simulink model "RobotX_ss_acoustics_1020"  (R2014a)
settings: Solver=FixedStepDiscrete  StartTime=0.0  StopTime=inf  FixedStep=.25  RelTol=1e-3
undefined symbols (not defined in the file): Com1, Com3, DiscIntNeverNeededParam, standard
libraries: xpcseriallib x19, dspmtrx3 x3, slrtlib x3, simulink x2, speedgoatlib x1, speedgoatlib_IO102 x1
(part 3 of 3)

== matlab function RobotX_ss_acoustics_1020/Main FSM/Acoustic FSM/Move 2/GPSMove ==
  data: GoalNED input; X input; Finished output; valid output; Y input; Psi input; pts output
function [Finished,valid,pts] = GPSmove(GoalNED,X,Y,Psi)
%Written by Dylan DeGaetano on September 1, 2014
%Last edited by: Anderson Lebbad
%
%This function will go to a given NED cooridnate, last edit changed the
%goal pt and variable names

persistent Sample
if isempty(Sample)
Sample = 0;
end
Finished = 0;
pts = zeros(8,2);
%$Distance to object in meters
if Sample >= 100
    Sample = 0;
end

if Sample == 0
    pts(1,1) = X+5*cos(Psi*pi/180);
    pts(1,2) = Y+5*cos(Psi*pi/180);
    pts(8,1) = GoalNED(1,1);
    pts(8,2) = GoalNED(1,2);
    pts(2,:) = pts(1,:) +(1*(GoalNED-pts(1,:))/7);
    pts(3,:) = pts(1,:) +(2*(GoalNED-pts(1,:))/7);
    pts(4,:) = pts(1,:) +(3*(GoalNED-pts(1,:))/7);
    pts(5,:) = pts(1,:) +(4*(GoalNED-pts(1,:))/7);
    pts(6,:) = pts(1,:) +(5*(GoalNED-pts(1,:))/7);
    pts(7,:) = pts(1,:) +(6*(GoalNED-pts(1,:))/7);
    Sample = 1; 
    valid = 1;
    
else 
    range = sqrt(sum((GoalNED - [X Y]).^2));
    if range <= 5
        Finished = 1;
    end
    valid = 0;
    Sample = Sample + 1;
end

== matlab function RobotX_ss_acoustics_1020/Main FSM/Acoustic FSM/Move 3/CalcTimes ==
  data: pts input; u input; Data output
function Data = calcTimes(pts, u)
%Written by Anderson Lebbad on August 9, 2014
%Last Edited: Dylan DeGaetano September 1, 2014

%Calculates times for the boat to get to points for a trajectory, and
%formats Data for communication

%Initialize
Data = zeros(24,1);
traj = zeros(8,3);
traj(:,1:2) = pts;



for k = 2:8
    %Calculate distance to travel from last point
    distTravel = sqrt(sum((pts(k-1,:)-pts(k,:)).^2));
    %Assume 1m per second speed
    traj(k,3) = traj(k-1,3) + distTravel;
    %Add time based off initial velocity to get to first point past initial
    if k == 2
        traj(k,3) = traj(k,3) + 2.5*abs(2-u);
    end
end


%Output Data
for i=1:8
    for j = 1:3
        Data(3*(i-1)+j) = traj(i,j);
    end
end

== matlab function RobotX_ss_acoustics_1020/Main FSM/Acoustic FSM/Move 3/GPSMove ==
  data: GoalNED input; X input; Finished output; valid output; Y input; Psi input; pts output
function [Finished,valid,pts] = GPSmove(GoalNED,X,Y,Psi)
%Written by Dylan DeGaetano on September 1, 2014
%Last edited by: Anderson Lebbad
%
%This function will go to a given NED cooridnate, last edit changed the
%goal pt and variable names

persistent Sample
if isempty(Sample)
Sample = 0;
end
Finished = 0;
pts = zeros(8,2);
%$Distance to object in meters
if Sample >= 100
    Sample = 0;
end

if Sample == 0
    pts(1,1) = X+5*cos(Psi*pi/180);
    pts(1,2) = Y+5*cos(Psi*pi/180);
    pts(8,1) = GoalNED(1,1);
    pts(8,2) = GoalNED(1,2);
    pts(2,:) = pts(1,:) +(1*(GoalNED-pts(1,:))/7);
    pts(3,:) = pts(1,:) +(2*(GoalNED-pts(1,:))/7);
    pts(4,:) = pts(1,:) +(3*(GoalNED-pts(1,:))/7);
    pts(5,:) = pts(1,:) +(4*(GoalNED-pts(1,:))/7);
    pts(6,:) = pts(1,:) +(5*(GoalNED-pts(1,:))/7);
    pts(7,:) = pts(1,:) +(6*(GoalNED-pts(1,:))/7);
    Sample = 1; 
    valid = 1;
    
else 
    range = sqrt(sum((GoalNED - [X Y]).^2));
    if range <= 5
        Finished = 1;
    end
    valid = 0;
    Sample = Sample + 1;
end

== matlab function RobotX_ss_acoustics_1020/Main FSM/Start//Speedgate/GPS Move/LLA to NED ==
  data: GoalLLA input; GoalNED output; NED_origin input
function GoalNED = LLA2NEDfun(GoalLLA,NED_origin)
%Written by Anderson Lebbad on September 20, 2014
%Last edited by:
%
%This function converts a target Latitude, Longitude, Altitude (LLA) point
%into North, East, Down (NED) coordinates

%First convert to earth centered, earth fixed frame
GoalECEF = lla2ecef([GoalLLA*(pi/180), 0]');
%Then convert from ECEF to North East Down
GoalNEDvect = ecef2ned(NED_origin'*(pi/180),GoalECEF);
GoalNED = GoalNEDvect(1:2)';

end

function x_ecef = lla2ecef(x_lla)
% LLE2ECEF: Converts from geodetic latitude, longitude, and altitude to earth-centered earth-fixed Cartesian coordinates
% INPUT: latitude phi (rad), longitude lambda (rad), altitude h (m)
% OUTPUT: [x, y, z]' (m) earth-centered earth-fixed Cartesian coordinates
    a = 6378137; % equatorial radius of ellipsoid (semi-major axis) (m)
    b = 6356752; % polar axis radius of ellipsoid (semi-minor axis) (m)

    phi = x_lla(1);
    lambda = x_lla(2);
    h = x_lla(3);
    
    % auxiliar quantities f, e, and N
    f = (a-b)/a;
    e = f*(2-f);
    N = a/sqrt(1-(e*sin(phi))^2);
    x_ecef = [(N+h)*cos(phi)*cos(lambda); (N+h)*cos(phi)*sin(lambda); (N*(1-e^2)+h)*sin(phi)];
end

function [x_ned] = ecef2ned(ned_lla, x_ecef)
% ECEF2NED Converts from earth-centered, earth-fixed Cartesian coordinates to tangent plane
% INPUT:
% 1) x_ecef=[x,y,z]' (m) earth-centered, earth-fixed Cartesian coordinates
% 2) ned_lla=[phi,lambda]' consiting of latitude phi (rad), longitude lambda (rad) of NED origin
% OUTPUT:
% 1) x_ned=[x,y,z]' (m) in NED coordinate system with the origin [phi,lambda]'

    phi = ned_lla(1);
    lambda = ned_lla(2);

    % transformation  matrix
    T = [-sin(phi)*cos(lambda) -sin(phi)*sin(lambda)  cos(phi)
         -sin(lambda)           cos(lambda)           0
          cos(phi)*cos(lambda)   cos(phi)*sin(lambda)  sin(phi)];

     x_ned = T*(x_ecef-lla2ecef([phi, lambda, 0]')); % convert to NED
     x_ned(3) = -x_ned(3);
end

== matlab function RobotX_ss_acoustics_1020/Sensors/Serial In/MATLAB Function3 ==
  data: Time input; asciiHRT output; Lat input; Long input; Mode input; Task input
% This function creates the heartbeat message to be sent from Speedgoat in
% ascii code
% Written by: Edward Zhu
% Date: 9/17/14

function asciiHRT = asciiHRTEncoder(Time, Lat, Long, Mode, Task)

% Initialize output message vector as the serial output block expects 128
% character message
asciiHRT = uint8(zeros(1,128));

% Convert static strings to ascii code
asciiMsgID = uint8('$RXHRT,');
asciiComma = uint8(',');
asciiDeciPt = uint8('.');
if Lat >= 0
    asciiNS = uint8('N,');
else
    Lat = -Lat;
    asciiNS = uint8('S,');
end
if Long >= 0
    asciiEW = uint8('E,');
else
    Long = -Long;
    asciiEW = uint8('W,');
end
asciiTeamID = uint8('FAUVU,');
asciiMsgEnd = uint8('*');
asciiMsgCRLF = [13 10];

% Convert UTC Time input (hhmmss) into ascii code
asciiTime = uint8(zeros(1,7));
asciiTime(7) = asciiComma;

for timeChar = 1:6
    asciiTime(timeChar) = floor(mod(Time,10^(7-timeChar))/...
        10^(6-timeChar)) + 48;
end

% Convert latitude (dd.mmmmmm) into ascii code
asciiLat = uint8(zeros(1,10));
asciiLat(10) = asciiComma;
asciiLat(3) = asciiDeciPt;

latInt = floor(Lat);
for latIntChar = 1:2
    asciiLat(latIntChar) = floor(mod(latInt,10^(3-latIntChar))/...
        10^(2-latIntChar)) + 48;
end

latDeci = mod(Lat,latInt) * 10^6;
for latDeciChar = 1:6
    asciiLat(latDeciChar+3) = floor(mod(latDeci,10^(7-latDeciChar))/...
        10^(6-latDeciChar)) + 48;
end

% Convert longitude (ddd.mmmmmm) into ascii code
asciiLong = uint8(zeros(1,11));
asciiLong(11) = asciiComma;
asciiLong(4) = asciiDeciPt;

longInt = floor(Long);
for longIntChar = 1:3
    asciiLong(longIntChar) = floor(mod(longInt,10^(4-longIntChar))/...
        10^(3-longIntChar)) + 48;
end

longDeci = mod(Long,longInt) * 10^6;
for longDeciChar = 1:6
    asciiLong(longDeciChar+4) = floor(mod(longDeci,10^(7-longDeciChar))/...
        10^(6-longDeciChar)) + 48;
end

% Convert vehicle mode into ascii (1 = RC, 2 = Auto)
if Mode ~= 1 || Mode ~= 2
    Mode = 1;
    asciiMode = [uint8(Mode+48) asciiComma];
else
    asciiMode = [uint8(Mode+48) asciiComma];
end

% Convert vehicle task into ascii
asciiTask = [uint8(Task+48) asciiMsgEnd];

% Concat individual ascii arrays into one array
asciiPreChkSum = cat(2,asciiMsgID,asciiTime,asciiLat,asciiNS,asciiLong,asciiEW,...
    asciiTeamID,asciiMode,asciiTask);

% Calculate the checksum of the message from the '$' to the '*' and convert
% to hex
chkSum = uint8(0);

for chksumChar = 1:(length(asciiPreChkSum)-2)
    chkSum = bitxor(chkSum,asciiPreChkSum(chksumChar+1));
end

% Convert the checksum to ascii
chkSum = dec2hex(chkSum);
asciiChkSum = uint8(zeros(1,length(chkSum))+32);
for i = 1:length(chkSum)
    asciiChkSum(i) = uint8(chkSum(i));
end

% Concat the checksum and the '/r/n' to the end of the message
asciiPostChkSum = cat(2,asciiPreChkSum,asciiChkSum,asciiMsgCRLF);

% Output the final message
asciiHRT(1:length(asciiPostChkSum)) = asciiPostChkSum;

== matlab function RobotX_ss_acoustics_1020/Sensors/Serial In/Data Update1 ==
  data: Valid input; ControlMode input; V output; C output; L output; A output; Data input; D1 output; D2 output; D3 output; D4 output; D5 output; D6 output; D7 output; D8 output; D9 output; D10 output; D11 output; D12 output; D13 output; D14 output; D15 output; D16 output; D17 output; D18 output; D19 output; D20 output; D21 output; D22 output; D23 output; D24 output; Activate input
function [V,C,L,A,D1,D2,D3,D4,D5,D6,D7,D8,D9,D10,D11,D12,D13,D14,D15,D16,D17,...
    D18,D19,D20,D21,D22,D23,D24] = dataSplit(Valid,ControlMode,Data,Activate)
%Written by Anderson Lebbad on August 10, 2014
%Last Edited by: Anderson Lebbad on September 11, 2014

%This function splits the data vector into the twelve channels it is
%composed of for communication

persistent HoldData

A = Activate;

if isempty(HoldData)
    HoldData = zeros(26,1);
end

L = 8;

if Valid == 1
    HoldData(1) = Valid;
    HoldData(2) = ControlMode;
    HoldData(3) = Data(1);
    HoldData(4) = Data(2);
    HoldData(5) = Data(3);
    HoldData(6) = Data(4);
    HoldData(7) = Data(5);
    HoldData(8) = Data(6);
    HoldData(9) = Data(7);
    HoldData(10) = Data(8);
    HoldData(11) = Data(9);
    HoldData(12) = Data(10);
    HoldData(13) = Data(11);
    HoldData(14) = Data(12);
    HoldData(15) = Data(13);
    HoldData(16) = Data(14);
    HoldData(17) = Data(15);
    HoldData(18) = Data(16);
    HoldData(19) = Data(17);
    HoldData(20) = Data(18);
    HoldData(21) = Data(19);
    HoldData(22) = Data(20);
    HoldData(23) = Data(21);
    HoldData(24) = Data(22);
    HoldData(25) = Data(23);
    HoldData(26) = Data(24);
end

V = HoldData(1);
C = HoldData(2);
D1 = HoldData(3);
D2 = HoldData(4);
D3 = HoldData(5);
D4 = HoldData(6);
D5 = HoldData(7);
D6 = HoldData(8);
D7 = HoldData(9);
D8 = HoldData(10);
D9 = HoldData(11);
D10 = HoldData(12);
D11 = HoldData(13);
D12 = HoldData(14);
D13 = HoldData(15);
D14 = HoldData(16);
D15 = HoldData(17);
D16 = HoldData(18);
D17 = HoldData(19);
D18 = HoldData(20);
D19 = HoldData(21);
D20 = HoldData(22);
D21 = HoldData(23);
D22 = HoldData(24);
D23 = HoldData(25);
D24 = HoldData(26);

end

== matlab function RobotX_ss_acoustics_1020/Main FSM/Acoustic FSM/Main Enabler ==
  data: taskSelector output; Drive1En output; Acoustic1En output; Drive2En output; Drive1Fin input; Acoustic1Fin input; Drive2Fin input; Acoustic2Fin input; Drive3Fin input; Acoustic3Fin input; Acoustic2En output; Drive3En output; Acoustic3En output; PointEn output
function [taskSelector,Drive1En,Acoustic1En,Drive2En,Acoustic2En,Drive3En,...
    Acoustic3En,PointEn] = taskEnabler(Drive1Fin,Acoustic1Fin,Drive2Fin,...
    Acoustic2Fin,Drive3Fin,Acoustic3Fin)
%Written by Anderson Lebbad on July 19, 2013
%Last Edited: Edward Zhu on June 2, 2014
%   Substring search for task was written in
%   Case switches were redundant, combined with first set of if statements

%Changes the value of MainMode and the enablers for the tasks within the
%Main FSM.

% Initialize enable signals
Drive1En = 0;
Acoustic1En = 0;
Drive2En = 0;
Acoustic2En = 0;
Drive3En = 0;
Acoustic3En = 0;
PointEn = 0;

% Set enable signals based on state completion
if Drive1Fin == 0
    Drive1En = 1;
    taskSelector = 1;
elseif Acoustic1Fin == 0
    Acoustic1En = 1;
    taskSelector = 2;
elseif Drive2Fin == 0
    Drive2En = 1;
    taskSelector = 3;
elseif Acoustic2Fin == 0
    Acoustic2En = 1;
    taskSelector = 4;
elseif Drive3Fin == 0
    Drive3En = 1;
    taskSelector = 5;
elseif Acoustic3Fin == 0
    Acoustic3En = 1;
    taskSelector = 6;
else
    PointEn = 1;
    taskSelector = 7;
end

== matlab function RobotX_ss_acoustics_1020/Main FSM/Acoustic FSM/Move 1/CalcTimes ==
  data: pts input; u input; Data output
function Data = calcTimes(pts, u)
%Written by Anderson Lebbad on August 9, 2014
%Last Edited: Dylan DeGaetano September 1, 2014

%Calculates times for the boat to get to points for a trajectory, and
%formats Data for communication

%Initialize
Data = zeros(24,1);
traj = zeros(8,3);
traj(:,1:2) = pts;



for k = 2:8
    %Calculate distance to travel from last point
    distTravel = sqrt(sum((pts(k-1,:)-pts(k,:)).^2));
    %Assume 1m per second speed
    traj(k,3) = traj(k-1,3) + distTravel;
    %Add time based off initial velocity to get to first point past initial
    if k == 2
        traj(k,3) = traj(k,3) + 2.5*abs(2-u);
    end
end


%Output Data
for i=1:8
    for j = 1:3
        Data(3*(i-1)+j) = traj(i,j);
    end
end

== matlab function RobotX_ss_acoustics_1020/Main FSM/Acoustic FSM/Move 1/GPSMove ==
  data: GoalNED input; X input; Finished output; valid output; Y input; Psi input; pts output
function [Finished,valid,pts] = GPSmove(GoalNED,X,Y,Psi)
%Written by Dylan DeGaetano on September 1, 2014
%Last edited by: Anderson Lebbad
%
%This function will go to a given NED cooridnate, last edit changed the
%goal pt and variable names

persistent Sample
if isempty(Sample)
Sample = 0;
end
Finished = 0;
pts = zeros(8,2);
%$Distance to object in meters
if Sample >= 100
    Sample = 0;
end

if Sample == 0
    pts(1,1) = X+5*cos(Psi*pi/180);
    pts(1,2) = Y+5*cos(Psi*pi/180);
    pts(8,1) = GoalNED(1,1);
    pts(8,2) = GoalNED(1,2);
    pts(2,:) = pts(1,:) +(1*(GoalNED-pts(1,:))/7);
    pts(3,:) = pts(1,:) +(2*(GoalNED-pts(1,:))/7);
    pts(4,:) = pts(1,:) +(3*(GoalNED-pts(1,:))/7);
    pts(5,:) = pts(1,:) +(4*(GoalNED-pts(1,:))/7);
    pts(6,:) = pts(1,:) +(5*(GoalNED-pts(1,:))/7);
    pts(7,:) = pts(1,:) +(6*(GoalNED-pts(1,:))/7);
    Sample = 1; 
    valid = 1;
    
else 
    range = sqrt(sum((GoalNED - [X Y]).^2));
    if range <= 5
        Finished = 1;
    end
    valid = 0;
    Sample = Sample + 1;
end

== matlab function RobotX_ss_acoustics_1020/Main FSM/Start//Speedgate/entrance/CalcTimes ==
  data: pts input; u input; Data output
function Data = calcTimes(pts, u)
%Written by Anderson Lebbad on August 9, 2014
%Last Edited: Dylan DeGaetano September 1, 2014

%Calculates times for the boat to get to points for a trajectory, and
%formats Data for communication

%Initialize
Data = zeros(24,1);
traj = zeros(8,3);
traj(:,1:2) = pts;



for k = 2:8
    %Calculate distance to travel from last point
    distTravel = sqrt(sum((pts(k-1,:)-pts(k,:)).^2));
    %Assume 1m per second speed
    traj(k,3) = traj(k-1,3) + distTravel;
    %Add time based off initial velocity to get to first point past initial
    if k == 2
        traj(k,3) = traj(k,3) + 2.5*abs(2-u);
    end
end


%Output Data
for i=1:8
    for j = 1:3
        Data(3*(i-1)+j) = traj(i,j);
    end
end

== matlab function RobotX_ss_acoustics_1020/Main FSM/Start//Speedgate/entrance/GPSMove ==
  data: GoalNED input; X input; Finished output; valid output; Y input; Psi input; pts output
function [Finished,valid,pts] = GPSmove(GoalNED,X,Y,Psi)
%Written by Dylan DeGaetano on September 1, 2014
%Last edited by: Anderson Lebbad
%
%This function will go to a given NED cooridnate, last edit changed the
%goal pt and variable names

persistent Sample
if isempty(Sample)
Sample = 0;
end
Finished = 0;
pts = zeros(8,2);
%$Distance to object in meters
if Sample >= 100
    Sample = 0;
end

if Sample == 0
    pts(1,1) = X+5*cos(Psi*pi/180);
    pts(1,2) = Y+5*cos(Psi*pi/180);
    pts(8,1) = GoalNED(1,1);
    pts(8,2) = GoalNED(1,2);
    pts(2,:) = pts(1,:) +(1*(GoalNED-pts(1,:))/7);
    pts(3,:) = pts(1,:) +(2*(GoalNED-pts(1,:))/7);
    pts(4,:) = pts(1,:) +(3*(GoalNED-pts(1,:))/7);
    pts(5,:) = pts(1,:) +(4*(GoalNED-pts(1,:))/7);
    pts(6,:) = pts(1,:) +(5*(GoalNED-pts(1,:))/7);
    pts(7,:) = pts(1,:) +(6*(GoalNED-pts(1,:))/7);
    Sample = 1; 
    valid = 1;
    
else 
    range = sqrt(sum((GoalNED - [X Y]).^2));
    if range <= 8
        Finished = 1;
    end
    valid = 0;
    Sample = Sample + 1;
end

== matlab function RobotX_ss_acoustics_1020/Main FSM/Start//Speedgate/exit/CalcTimes ==
  data: pts input; u input; Data output
function Data = calcTimes(pts, u)
%Written by Anderson Lebbad on August 9, 2014
%Last Edited: Dylan DeGaetano September 1, 2014

%Calculates times for the boat to get to points for a trajectory, and
%formats Data for communication

%Initialize
Data = zeros(24,1);
traj = zeros(8,3);
traj(:,1:2) = pts;



for k = 2:8
    %Calculate distance to travel from last point
    distTravel = sqrt(sum((pts(k-1,:)-pts(k,:)).^2));
    %Assume 1m per second speed
    traj(k,3) = traj(k-1,3) + distTravel;
    %Add time based off initial velocity to get to first point past initial
    if k == 2
        traj(k,3) = traj(k,3) + 2.5*abs(2-u);
    end
end


%Output Data
for i=1:8
    for j = 1:3
        Data(3*(i-1)+j) = traj(i,j);
    end
end

== matlab function RobotX_ss_acoustics_1020/Main FSM/Start//Speedgate/exit/GPSMove ==
  data: GoalNED input; X input; Finished output; valid output; Y input; Psi input; pts output
function [Finished,valid,pts] = GPSmove(GoalNED,X,Y,Psi)
%Written by Dylan DeGaetano on September 1, 2014
%Last edited by: Anderson Lebbad
%
%This function will go to a given NED cooridnate, last edit changed the
%goal pt and variable names

persistent Sample
if isempty(Sample)
Sample = 0;
end
Finished = 0;
pts = zeros(8,2);
%$Distance to object in meters
if Sample >= 100
    Sample = 0;
end

if Sample == 0
    pts(1,1) = X+5*cos(Psi*pi/180);
    pts(1,2) = Y+5*cos(Psi*pi/180);
    pts(8,1) = GoalNED(1,1);
    pts(8,2) = GoalNED(1,2);
    pts(2,:) = pts(1,:) +(1*(GoalNED-pts(1,:))/7);
    pts(3,:) = pts(1,:) +(2*(GoalNED-pts(1,:))/7);
    pts(4,:) = pts(1,:) +(3*(GoalNED-pts(1,:))/7);
    pts(5,:) = pts(1,:) +(4*(GoalNED-pts(1,:))/7);
    pts(6,:) = pts(1,:) +(5*(GoalNED-pts(1,:))/7);
    pts(7,:) = pts(1,:) +(6*(GoalNED-pts(1,:))/7);
    Sample = 1; 
    valid = 1;
    
else 
    range = sqrt(sum((GoalNED - [X Y]).^2));
    if range <= 8
        Finished = 1;
    end
    valid = 0;
    Sample = Sample + 1;
end

== matlab function RobotX_ss_acoustics_1020/Main FSM/Termination/CalcTimes ==
  data: pts input; u input; Data output
function Data = calcTimes(pts, u)
%Written by Anderson Lebbad on August 9, 2014
%Last Edited: Dylan DeGaetano September 1, 2014

%Calculates times for the boat to get to points for a trajectory, and
%formats Data for communication

%Initialize
Data = zeros(24,1);
traj = zeros(8,3);
traj(:,1:2) = pts;



for k = 2:8
    %Calculate distance to travel from last point
    distTravel = sqrt(sum((pts(k-1,:)-pts(k,:)).^2));
    %Assume 1m per second speed
    traj(k,3) = traj(k-1,3) + distTravel;
    %Add time based off initial velocity to get to first point past initial
    if k == 2
        traj(k,3) = traj(k,3) + 2.5*abs(2-u);
    end
end


%Output Data
for i=1:8
    for j = 1:3
        Data(3*(i-1)+j) = traj(i,j);
    end
end

== matlab function RobotX_ss_acoustics_1020/Main FSM/Termination/GPSMove ==
  data: GoalNED input; X input; valid output; Y input; Psi input; pts output
function [valid,pts] = GPSmove(GoalNED,X,Y,Psi)
%Written by Dylan DeGaetano on September 1, 2014
%Last edited by: Anderson Lebbad
%
%This function will go to a given NED cooridnate, last edit changed the
%goal pt and variable names

persistent Sample
if isempty(Sample)
Sample = 0;
end

pts = zeros(8,2);
%$Distance to object in meters

if Sample == 0
    pts(1,1) = X+5*cos(Psi*pi/180);
    pts(1,2) = Y+5*cos(Psi*pi/180);
    pts(8,1) = GoalNED(1,1);
    pts(8,2) = GoalNED(1,2);
    pts(2,:) = pts(1,:) +(1*(GoalNED-pts(1,:))/7);
    pts(3,:) = pts(1,:) +(2*(GoalNED-pts(1,:))/7);
    pts(4,:) = pts(1,:) +(3*(GoalNED-pts(1,:))/7);
    pts(5,:) = pts(1,:) +(4*(GoalNED-pts(1,:))/7);
    pts(6,:) = pts(1,:) +(5*(GoalNED-pts(1,:))/7);
    pts(7,:) = pts(1,:) +(6*(GoalNED-pts(1,:))/7);
    Sample = 1; 
    valid = 1;
    
else
    valid = 0;
end
